simulink model "pada_plant_model_testing"  (R2022b)
settings: Solver=VariableStepAuto  StartTime=0.0  StopTime=20  RelTol=1e-3
values from neighbouring files (symbols this model uses):
  A_lon = [du_u,  du_w,   du_q,   du_theta ... (first row only)    [pada_linear_model.m]
  B_lon = [du_de,     du_dt ... (first row only)    [pada_linear_model.m]
  C_D0 = 0.0159    [pada_aero_coefficients.m]
  C_Dalpha = 0    [pada_aero_coefficients.m]
  C_Dde = 0    [pada_aero_coefficients.m]
  C_Dq = 0    [pada_aero_coefficients.m]
  C_l0 = 0.0033    [pada_aero_coefficients.m]
  C_L0 = 0.0193    [pada_aero_coefficients.m]
  C_Lalpha = 0.056    [pada_aero_coefficients.m]
  C_lbeta = -0.04415    [pada_aero_coefficients.m]
  C_lda = 0.0025326    [pada_aero_coefficients.m]
  C_Lde = 0    [pada_aero_coefficients.m]
  C_lon = eye(4)    [pada_linear_model.m]
  C_Lq = 3.48391    [pada_aero_coefficients.m]
  C_m0 = 0.00045    [pada_aero_coefficients.m]
  C_malpha = -0.3787    [pada_aero_coefficients.m]
  C_mde = 0    [pada_aero_coefficients.m]
  C_mq = -1.26832    [pada_aero_coefficients.m]
  C_n0 = 0    [pada_aero_coefficients.m]
  C_nbeta = 0.12637    [pada_aero_coefficients.m]
  C_nda = 0    [pada_aero_coefficients.m]
  C_Xde = C_Xde    [pada_linear_model.m]
  C_Y0 = 0    [pada_aero_coefficients.m]
  C_Ybeta = -0.6377    [pada_aero_coefficients.m]
  C_Yda = 0    [pada_aero_coefficients.m]
  C_Yp = -0.06787    [pada_aero_coefficients.m]
  C_Yr = 0.51996    [pada_aero_coefficients.m]
  C_Zde = C_Zde    [pada_linear_model.m]
  D_lon = zeros(4,2)    [pada_linear_model.m]
  g = 9.81    [pada_plant.m]
  J_x = 1    [pada_plant.m]
  J_xz = 1    [pada_plant.m]
  J_y = 1    [pada_plant.m]
  J_z = 1    [pada_plant.m]
  k_motor = 1    [pada_plant.m]
  m = 1    [pada_plant.m]
  q_0 = 0    [pada_linear_model.m]
  Ref_area = 1    [pada_plant.m]
  Ref_chord = 1    [pada_plant.m]
  Ref_span = 1    [pada_plant.m]
  rho = 1    [pada_plant.m]
  S_prop = 1    [pada_plant.m]
  theta_0 = 0.01    [pada_linear_model.m]
  u_0 = 10.0    (= 10)    [pada_linear_model.m]
  w_0 = 1.0    (= 1)    [pada_linear_model.m]
undefined symbols (not defined in the file or in its folder): C_Xda, C_Zda, K_lon
libraries: simulink_extras x5, slpidlib x4, shared6dof x3, aerolibasang x3, sharedtransform x1, uavutilslib x1
(part 2 of 2)

== system pada_plant_model_testing/Plant3/Aerodynamics/Forces and Moments ==
  Coef_stab : Inport
  AoA : Inport  Port=2
  Va : Inport  Port=3
  Constant : Constant  Value=rho
  Constant1 : Constant  Value=Ref_area
  Constant2 : Constant  Value=Ref_span
  Constant3 : Constant  Value=Ref_chord
  MATLAB Function1 : MATLAB Function  TreatAsAtomicUnit=on
  F_aero : Outport
  M_aero : Outport  Port=2
  wires:
  Constant3/1 -> MATLAB Function1/7(Ref_chord)
  Va/1 -> MATLAB Function1/3(Va)
  Constant1/1 -> MATLAB Function1/5(Ref_area)
  Constant/1 -> MATLAB Function1/4(rho)
  Coef_stab/1 -> MATLAB Function1/1(Coef_stab)
  AoA/1 -> MATLAB Function1/2(AoA)
  Constant2/1 -> MATLAB Function1/6(Ref_span)
  MATLAB Function1/1(F_aero) -> F_aero/1
  MATLAB Function1/2(M_aero) -> M_aero/1

== matlab function pada_plant_model_testing/Plant1/Gravity/MATLAB Function1 ==
  data: pitch input; F_grav output; roll input; m input; g input
function F_grav = GravityInBody(pitch, roll, m, g)

F_gx = -m*g*sin(pitch);
F_gy = m*g*cos(pitch)*sin(roll);
F_gz = m*g*cos(pitch)*cos(roll);

F_grav = [F_gx, F_gy, F_gz];

== matlab function pada_plant_model_testing/Plant1/Propulsion/MATLAB Function1 ==
  data: Thr input; F_prop output; Va input; rho input; S_prop input; k_motor input
function F_prop = ForcePropInBody(Thr, Va, rho, S_prop, k_motor)

F_xp = 0.5 * rho * S_prop * ((k_motor * Thr)^2 - Va^2);
F_prop = [F_xp, 0, 0];

== matlab function pada_plant_model_testing/Plant3/Aerodynamics/Aero Coefficients/MATLAB Function2 ==
  data: AoA input; SSA input; Coef_stab output; Ele input; Ail input; C_D_coeff input; C_Y_coeff input; C_L_coeff input; C_l_coeff input; C_m_coeff input; C_n_coeff input; C_de_coeff input; C_da_coeff input
function Coef_stab = AeroCoef(AoA, SSA, Ele, Ail, C_D_coeff, C_Y_coeff, C_L_coeff, C_l_coeff, C_m_coeff, C_n_coeff, C_de_coeff, C_da_coeff)

C_D0 = C_D_coeff(1);
C_Dalpha = C_D_coeff(2);
%C_Dq = C_D_coeff(3);
%C_Dde = C_D_coeff(4);

C_Y0 = C_Y_coeff(1);
C_Ybeta = C_Y_coeff(2);
%C_Yp = C_Y_coeff(3);
%C_Yr = C_Y_coeff(4);
C_Yda = C_Y_coeff(5);

C_L0 = C_L_coeff(1);
C_Lalpha = C_L_coeff(2);
%C_Lq = C_L_coeff(3);
%C_Lde = C_L_coeff(4);

C_l0 = C_l_coeff(1);
C_lbeta = C_l_coeff(2);
C_lda = C_l_coeff(3);

C_m0 = C_m_coeff(1);
C_malpha = C_m_coeff(2);
%C_mq = C_m_coeff(3);
C_mde = C_m_coeff(4);

C_n0 = C_n_coeff(1);
C_nbeta = C_n_coeff(2);
C_nda = C_n_coeff(3);

C_Xde = C_de_coeff(1);
C_Zde = C_de_coeff(2);

%C_Xda = C_da_coeff(1);
%C_Zda = C_da_coeff(2);

C_Dde = -C_Xde*cos(AoA) - C_Zde*sin(AoA);
C_Lde = C_Xde*sin(AoA) - C_Zde*cos(AoA);

% F_x = -F_drag * cos(AoA) + F_lift * sin(AoA);
% F_y = factor * C_y;
% F_z = -F_drag * sin(AoA) - F_lift * cos(AoA);

C_D = C_D0 + C_Dalpha * AoA + C_Dde * Ele;
C_Y = C_Y0 + C_Ybeta * SSA + C_Yda * Ail;
C_L = C_L0 + C_Lalpha * AoA + C_Lde * Ele;
C_l = C_l0 + C_lbeta * SSA + C_lda * Ail;
C_m = C_m0 + C_malpha * AoA + C_mde * Ele;
C_n = C_n0 + C_nbeta * SSA + C_nda * Ail;

Coef_stab = [C_D, C_Y, C_L, C_l, C_m, C_n];

== matlab function pada_plant_model_testing/Plant3/Aerodynamics/Forces and Moments/MATLAB Function1 ==
  data: Coef_stab input; AoA input; F_aero output size=[1 3]; M_aero output size=[1 3]; Va input; rho input; Ref_area input; Ref_span input; Ref_chord input
function [F_aero, M_aero]= AeroForcesInBody(Coef_stab, AoA, Va, rho, Ref_area, Ref_span, Ref_chord)

C_D = Coef_stab(1);
C_y = Coef_stab(2);
C_L = Coef_stab(3);
C_l = Coef_stab(4);
C_m = Coef_stab(5);
C_n = Coef_stab(6);

factor = 0.5*rho*Va*Va*Ref_area;

F_lift = factor * C_L;
F_drag = factor * C_D;
F_x = -F_drag * cos(AoA) + F_lift * sin(AoA);
F_y = factor * C_y;
F_z = -F_drag * sin(AoA) - F_lift * cos(AoA);

l = factor * Ref_span * C_l;
m = factor * Ref_chord * C_m;
n = factor * Ref_span * C_n;

F_aero = [F_x, F_y, F_z];
M_aero = [l, m, n];

== matlab function pada_plant_model_testing/Plant3/Gravity/MATLAB Function1 ==
  data: pitch input; F_grav output; roll input; m input; g input
function F_grav = GravityInBody(pitch, roll, m, g)

F_gx = -m*g*sin(pitch);
F_gy = m*g*cos(pitch)*sin(roll);
F_gz = m*g*cos(pitch)*cos(roll);

F_grav = [F_gx, F_gy, F_gz];

== matlab function pada_plant_model_testing/Plant3/Propulsion/MATLAB Function1 ==
  data: Thr input; F_prop output; Va input; rho input; S_prop input; k_motor input
function F_prop = ForcePropInBody(Thr, Va, rho, S_prop, k_motor)

F_xp = 0.5 * rho * S_prop * ((k_motor * Thr)^2 - Va^2);
F_prop = [F_xp, 0, 0];

== matlab function pada_plant_model_testing/MATLAB Function ==
  data: u input; h_dot output; w input; theta input
function h_dot = delta_h(u, w, theta)

h_dot = u*sin(theta) - w*cos(theta);

== matlab function pada_plant_model_testing/Plant2/Aerodynamics/Aero Coefficients/MATLAB Function2 ==
  data: AoA input; SSA input; Coef_stab output; Ele input; Ail input; C_D_coeff input; C_Y_coeff input; C_L_coeff input; C_l_coeff input; C_m_coeff input; C_n_coeff input; C_de_coeff input; C_da_coeff input
function Coef_stab = AeroCoef(AoA, SSA, Ele, Ail, C_D_coeff, C_Y_coeff, C_L_coeff, C_l_coeff, C_m_coeff, C_n_coeff, C_de_coeff, C_da_coeff)

C_D0 = C_D_coeff(1);
C_Dalpha = C_D_coeff(2);
%C_Dq = C_D_coeff(3);
%C_Dde = C_D_coeff(4);

C_Y0 = C_Y_coeff(1);
C_Ybeta = C_Y_coeff(2);
%C_Yp = C_Y_coeff(3);
%C_Yr = C_Y_coeff(4);
C_Yda = C_Y_coeff(5);

C_L0 = C_L_coeff(1);
C_Lalpha = C_L_coeff(2);
%C_Lq = C_L_coeff(3);
%C_Lde = C_L_coeff(4);

C_l0 = C_l_coeff(1);
C_lbeta = C_l_coeff(2);
C_lda = C_l_coeff(3);

C_m0 = C_m_coeff(1);
C_malpha = C_m_coeff(2);
%C_mq = C_m_coeff(3);
C_mde = C_m_coeff(4);

C_n0 = C_n_coeff(1);
C_nbeta = C_n_coeff(2);
C_nda = C_n_coeff(3);

C_Xde = C_de_coeff(1);
C_Zde = C_de_coeff(2);

%C_Xda = C_da_coeff(1);
%C_Zda = C_da_coeff(2);

C_Dde = -C_Xde*cos(AoA) - C_Zde*sin(AoA);
C_Lde = C_Xde*sin(AoA) - C_Zde*cos(AoA);

% F_x = -F_drag * cos(AoA) + F_lift * sin(AoA);
% F_y = factor * C_y;
% F_z = -F_drag * sin(AoA) - F_lift * cos(AoA);

C_D = C_D0 + C_Dalpha * AoA + C_Dde * Ele;
C_Y = C_Y0 + C_Ybeta * SSA + C_Yda * Ail;
C_L = C_L0 + C_Lalpha * AoA + C_Lde * Ele;
C_l = C_l0 + C_lbeta * SSA + C_lda * Ail;
C_m = C_m0 + C_malpha * AoA + C_mde * Ele;
C_n = C_n0 + C_nbeta * SSA + C_nda * Ail;

Coef_stab = [C_D, C_Y, C_L, C_l, C_m, C_n];

== matlab function pada_plant_model_testing/MATLAB Function2 ==
  data: u input; h_dot output; w input; theta input
function h_dot = delta_h(u, w, theta)

h_dot = u*sin(theta) - w*cos(theta);

== matlab function pada_plant_model_testing/MATLAB Function1 ==
  data: u input; va output; w input
function va = arspd(u,w)

va = sqrt(u^2 + w^2);

== matlab function pada_plant_model_testing/Plant2/Aerodynamics/Forces and Moments/MATLAB Function1 ==
  data: Coef_stab input; AoA input; F_aero output size=[1 3]; M_aero output size=[1 3]; Va input; rho input; Ref_area input; Ref_span input; Ref_chord input
function [F_aero, M_aero]= AeroForcesInBody(Coef_stab, AoA, Va, rho, Ref_area, Ref_span, Ref_chord)

C_D = Coef_stab(1);
C_y = Coef_stab(2);
C_L = Coef_stab(3);
C_l = Coef_stab(4);
C_m = Coef_stab(5);
C_n = Coef_stab(6);

factor = 0.5*rho*Va*Va*Ref_area;

F_lift = factor * C_L;
F_drag = factor * C_D;
F_x = -F_drag * cos(AoA) + F_lift * sin(AoA);
F_y = factor * C_y;
F_z = -F_drag * sin(AoA) - F_lift * cos(AoA);

l = factor * Ref_span * C_l;
m = factor * Ref_chord * C_m;
n = factor * Ref_span * C_n;

F_aero = [F_x, F_y, F_z];
M_aero = [l, m, n];

== matlab function pada_plant_model_testing/Plant2/Gravity/MATLAB Function1 ==
  data: pitch input; F_grav output; roll input; m input; g input
function F_grav = GravityInBody(pitch, roll, m, g)

F_gx = -m*g*sin(pitch);
F_gy = m*g*cos(pitch)*sin(roll);
F_gz = m*g*cos(pitch)*cos(roll);

F_grav = [F_gx, F_gy, F_gz];

== matlab function pada_plant_model_testing/Plant1/Aerodynamics/Aero Coefficients/MATLAB Function2 ==
  data: AoA input; SSA input; Coef_stab output; Ele input; Ail input; C_D_coeff input; C_Y_coeff input; C_L_coeff input; C_l_coeff input; C_m_coeff input; C_n_coeff input; C_de_coeff input; C_da_coeff input
function Coef_stab = AeroCoef(AoA, SSA, Ele, Ail, C_D_coeff, C_Y_coeff, C_L_coeff, C_l_coeff, C_m_coeff, C_n_coeff, C_de_coeff, C_da_coeff)

C_D0 = C_D_coeff(1);
C_Dalpha = C_D_coeff(2);
%C_Dq = C_D_coeff(3);
%C_Dde = C_D_coeff(4);

C_Y0 = C_Y_coeff(1);
C_Ybeta = C_Y_coeff(2);
%C_Yp = C_Y_coeff(3);
%C_Yr = C_Y_coeff(4);
C_Yda = C_Y_coeff(5);

C_L0 = C_L_coeff(1);
C_Lalpha = C_L_coeff(2);
%C_Lq = C_L_coeff(3);
%C_Lde = C_L_coeff(4);

C_l0 = C_l_coeff(1);
C_lbeta = C_l_coeff(2);
C_lda = C_l_coeff(3);

C_m0 = C_m_coeff(1);
C_malpha = C_m_coeff(2);
%C_mq = C_m_coeff(3);
C_mde = C_m_coeff(4);

C_n0 = C_n_coeff(1);
C_nbeta = C_n_coeff(2);
C_nda = C_n_coeff(3);

C_Xde = C_de_coeff(1);
C_Zde = C_de_coeff(2);

%C_Xda = C_da_coeff(1);
%C_Zda = C_da_coeff(2);

C_Dde = -C_Xde*cos(AoA) - C_Zde*sin(AoA);
C_Lde = C_Xde*sin(AoA) - C_Zde*cos(AoA);

% F_x = -F_drag * cos(AoA) + F_lift * sin(AoA);
% F_y = factor * C_y;
% F_z = -F_drag * sin(AoA) - F_lift * cos(AoA);

C_D = C_D0 + C_Dalpha * AoA + C_Dde * Ele;
C_Y = C_Y0 + C_Ybeta * SSA + C_Yda * Ail;
C_L = C_L0 + C_Lalpha * AoA + C_Lde * Ele;
C_l = C_l0 + C_lbeta * SSA + C_lda * Ail;
C_m = C_m0 + C_malpha * AoA + C_mde * Ele;
C_n = C_n0 + C_nbeta * SSA + C_nda * Ail;

Coef_stab = [C_D, C_Y, C_L, C_l, C_m, C_n];

== matlab function pada_plant_model_testing/Plant2/Propulsion/MATLAB Function1 ==
  data: Thr input; F_prop output; Va input; rho input; S_prop input; k_motor input
function F_prop = ForcePropInBody(Thr, Va, rho, S_prop, k_motor)

F_xp = 0.5 * rho * S_prop * ((k_motor * Thr)^2 - Va^2);
F_prop = [F_xp, 0, 0];

== matlab function pada_plant_model_testing/Plant1/Aerodynamics/Forces and Moments/MATLAB Function1 ==
  data: Coef_stab input; AoA input; F_aero output size=[1 3]; M_aero output size=[1 3]; Va input; rho input; Ref_area input; Ref_span input; Ref_chord input
function [F_aero, M_aero]= AeroForcesInBody(Coef_stab, AoA, Va, rho, Ref_area, Ref_span, Ref_chord)

C_D = Coef_stab(1);
C_y = Coef_stab(2);
C_L = Coef_stab(3);
C_l = Coef_stab(4);
C_m = Coef_stab(5);
C_n = Coef_stab(6);

factor = 0.5*rho*Va*Va*Ref_area;

F_lift = factor * C_L;
F_drag = factor * C_D;
F_x = -F_drag * cos(AoA) + F_lift * sin(AoA);
F_y = factor * C_y;
F_z = -F_drag * sin(AoA) - F_lift * cos(AoA);

l = factor * Ref_span * C_l;
m = factor * Ref_chord * C_m;
n = factor * Ref_span * C_n;

F_aero = [F_x, F_y, F_z];
M_aero = [l, m, n];
